simulink model "suspmod"  (R2018b)
settings: Solver=ode45  StartTime=0.0  StopTime=50  RelTol=1e-3  AbsTol=1e-6
settings Model: Creator=Konish  LastModifiedBy=Konish
settings DataIOCC: SaveFormat=Array  SignalLoggingSaveFormat=ModelDataLogs
settings OptimizationCC: BlockReduction=off  BooleanDataType=off
settings DebuggingCC: SaveWithParameterizedLinksMsg=none  UnderspecifiedInitializationDetection=Classic  MergeDetectMultiDrivingBlocksExec=none  SignalResolutionControl=TryResolveAllWithWarning  MultiTaskDSMMsg=warning  MultiTaskCondExecSysMsg=none
settings HardwareCC: TargetUnknown=on
settings ModelReferenceCC: PropagateSignalLabelsOutOfModel=off

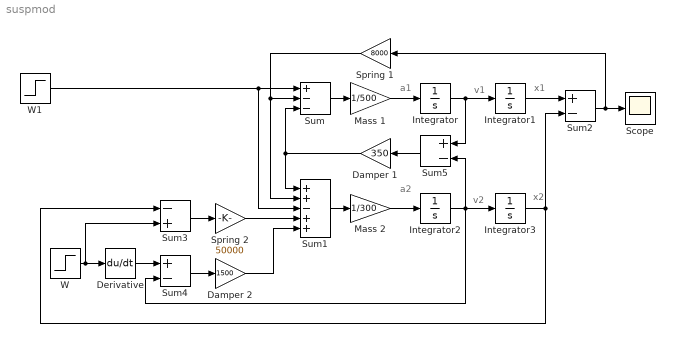
== system suspmod ==
  note: a1
  note: v1
  note: x1
  note: a2
  note: v2
  note: x2
  Damper 1 : Gain  Gain=350  SaturateOnIntegerOverflow=on  OutDataTypeStr=Inherit: Same as input  ParamDataTypeStr=Inherit: Same as input
  Damper 2 : Gain  Gain=1500  SaturateOnIntegerOverflow=on  OutDataTypeStr=Inherit: Same as input  ParamDataTypeStr=Inherit: Same as input
  Derivative : Derivative
  Integrator{,1..3} (4 alike) : Integrator
  Mass 1 : Gain  Gain=1/500  SaturateOnIntegerOverflow=on  OutDataTypeStr=Inherit: Same as input  ParamDataTypeStr=Inherit: Same as input
  Mass 2 : Gain  Gain=1/300  SaturateOnIntegerOverflow=on  OutDataTypeStr=Inherit: Same as input  ParamDataTypeStr=Inherit: Same as input
  Scope : Scope
  Spring 1 : Gain  Gain=8000  SaturateOnIntegerOverflow=on  OutDataTypeStr=Inherit: Same as input  ParamDataTypeStr=Inherit: Same as input
  Spring 2 : Gain  Gain=50000  SaturateOnIntegerOverflow=on  OutDataTypeStr=Inherit: Same as input  ParamDataTypeStr=Inherit: Same as input
  Sum : Sum  Inputs=+--  SaturateOnIntegerOverflow=on  InputSameDT=on  OutDataTypeStr=Inherit: Same as first input
  Sum1 : Sum  Inputs=++-++  SaturateOnIntegerOverflow=on  InputSameDT=on  OutDataTypeStr=Inherit: Same as first input
  Sum2 : Sum  Inputs=+-  SaturateOnIntegerOverflow=on  InputSameDT=on  OutDataTypeStr=Inherit: Same as first input
  Sum3 : Sum  Inputs=-+  SaturateOnIntegerOverflow=on  InputSameDT=on  OutDataTypeStr=Inherit: Same as first input
  Sum4 : Sum  Inputs=+-  SaturateOnIntegerOverflow=on  InputSameDT=on  OutDataTypeStr=Inherit: Same as first input
  Sum5 : Sum  Inputs=+-  SaturateOnIntegerOverflow=on  InputSameDT=on  OutDataTypeStr=Inherit: Same as first input
  W : Step  Time=0  SampleTime=0
  W1 : Step  Time=0  SampleTime=0
  wires:
  Mass 2/1 -> Integrator2/1
  Sum1/1 -> Mass 2/1
  Integrator2/1 -> Integrator3/1, Sum4/2, Sum5/2
  Sum5/1 -> Damper 1/1
  Damper 1/1 -> Sum/3, Sum1/1
  Mass 1/1 -> Integrator/1
  Sum/1 -> Mass 1/1
  Integrator1/1 -> Sum2/1
  Integrator/1 -> Integrator1/1, Sum5/1
  Integrator3/1 -> Sum2/2, Sum3/1
  Sum2/1 -> Scope/1, Spring 1/1
  Spring 1/1 -> Sum/2, Sum1/2
  Sum3/1 -> Spring 2/1
  Sum4/1 -> Damper 2/1
  W1/1 -> Sum1/3, Sum/1
  Derivative/1 -> Sum4/1
  W/1 -> Sum3/2, Derivative/1
  Damper 2/1 -> Sum1/5
  Spring 2/1 -> Sum1/4
